simulink model "IDTmodel"  (R2021a)
settings: Solver=ode23tb  StartTime=0.0  StopTime=0.75  FixedStep=4e-4  RelTol=1e-3  EnableMultiTasking=on
PreLoadFcn:
  | % -- Recommended Settings --
  | %
  | %  Simulink:
  | %      Solver: Ode23tb
  | %      Relative tolerance = 1e-4
  | %      Max step size = 0.2
  | %
  | %  Powergui:
  |          Ts = 1e-06; % (discrete electrical model)
  | %
  | %  Control systems:
  |          Ts_control = 10*Ts; % (discrete control system)
  | %
  | % ----------------------------------
InitFcn:
  | Ts=1e-5;
  | Ts_control=1e-5;
undefined symbols (not defined in the file or in its folder): D1, Delta
libraries: spsThreePhaseVIMeasurementLib x26, spsThreePhaseSeriesRLCLoadLib x8, spsabctoAlphaBetaZeroLib x6, spsThreePhaseSeriesRLCBranchLib x6, spsThreePhaseTransformerTwoWindingsLib x5, spsDistributedParametersLineLib x5, spsPowerPositiveSequenceLib x4, spsThreePhaseBreakerLib x4, spsDCVoltageSourceLib x2, spsSVPWMGenerator2LevelLib x2, spsGroundLib x2, spsUniversalBridgeLib x2
(part 2 of 2)

== system IDTmodel/DL-5 ==
  20Km feeder : spsDistributedParametersLineLib/Distributed Parameters Line  Phases=3  Length=20  Frequency=50  Resistance=[0.1153 0.413]  Inductance=[1.05e-3 3.32e-3]  Capacitance=[11.33e-009 5.01e-009]  x1=[-9e-05 -1.85671820461914e-09 0 0;-8e-05 -1.85401382529522e-09 0 0;-7e-05 -1.85129114760334e-09 20803.2327751115 -13139.8661984527;-6e-05 -1.84855019841523e-09 20844.4101545723 -13074.4461801133;-5e-05 -1.84579100478295e-09 20885.3818081202 -13008.8971222685;-4e-05 -1.84301359393864e-09 20926.1473313813 -12943.219671861;-3e-05 -1.8402179932942e-09 20966.7063220166 -12877.4144771007;-2e-05 -1.8374042304411e-09 21007.058379725 -12811.4821874584;-1e-05 -1.83457233315003e-09 21047.2031062481 -12745.4234536591]  x2=[-9e-05 -1.69133325708034e-10 0 0;-8e-05 -1.69244704148608e-10 0 0;-7e-05 -1.69354412212279e-10 20557.5369180313 -13274.4665234826;-6e-05 -1.69462448816273e-10 20599.1383686483 -13209.8177159477;-5e-05 -1.69568812894312e-10 20640.5365140858 -13145.038532845;-4e-05 -1.69673503396625e-10 20681.7309457608 -13080.1296135189;-3e-05 -1.69776519289959e-10 20722.721257101 -13015.0915985941;-2e-05 -1.6987785955759e-10 20763.5070435485 -12949.9251299696;-1e-05 -1.6997752319933e-10 20804.087902564 -12884.6308508122]  x3=[-9e-05 6.18585301934319e-11 0 0;-8e-05 6.20328462935421e-11 0 0;-7e-05 6.22065501545031e-11 37.8134386631987 -16.9223687566623;-6e-05 6.2379640061928e-11 37.8664151634293 -16.8034910224862;-5e-05 6.2552114307489e-11 37.9190179374296 -16.6844474446375;-4e-05 6.27239711889352e-11 37.9712464660314 -16.5652391980283;-3e-05 6.28952090101084e-11 38.0231002337601 -16.4458674591959;-2e-05 6.30658260809605e-11 38.0745787288401 -16.3263334062911;-1e-05 6.32358207175699e-11 38.1256814431994 -16.2066382190668]  x4=[-9e-05 -6.47056572877299e-11 0 0;-8e-05 -6.48780349176388e-11 0 0;-7e-05 -6.50497722275354e-11 96.345814689957 -70.8209858434872;-6e-05 -6.52208675224418e-11 96.5678295656737 -70.5179575504712;-5e-05 -6.53913191137165e-11 96.7888913558986 -70.2142332736835;-4e-05 -6.5561125319071e-11 97.008997878841 -69.9098160107601;-3e-05 -6.57302844625868e-11 97.2281469621385 -69.6047087661763;-2e-05 -6.58987948747313e-11 97.4463364428781 -69.2989145512176;-1e-05 -6.60666548923748e-11 97.6635641676177 -68.9924363839494]  x5=8.1567640642598e-05  V1=[0 0 0 1.943e-09 2.476e+04 2.476e+04;0 0 0 314.2 314.2 314.2;1.571 1.571 1.571 2.213 1.006 -0.5651]  V2=[0 0 0 8.204e-11 2.462e+04 2.462e+04;0 0 0 314.2 314.2 314.2;1.571 1.571 1.571 -1.53 0.9957 -0.5751]  I1=[0 0 0 8.843e-11 41.68 41.68;0 0 0 314.2 314.2 314.2;1.571 1.571 1.571 -2.172 1.148 -0.4225]  I2=[0 0 0 8.932e-11 120.3 120.3;0 0 0 314.2 314.2 314.2;1.571 1.571 1.571 1.001 0.9352 -0.6356]  nHarmo=2  Measurements=None  Decoupling=off  VsMag0=0  VrMag0=0  VsAngle0=0  VrAngle0=0  IsMag0=0  IrMag0=0  IsAngle0=0  IrAngle0=0
      settings: SourceProductBaseCode=PS
  Three-Phase V-I Measurement1 : spsThreePhaseVIMeasurementLib/Three-Phase V-I Measurement  VoltageMeasurement=no  SetLabelV=off  LabelV=Vabc  Vpu=on  VpuLL=off  CurrentMeasurement=no  SetLabelI=off  LabelI=I23  Ipu=on  Pbase=6e6  Vbase=12.47e3  OutputType=Complex  PhasorSimulation=off  PSBequivalent=0
  Three-Phase V-I Measurement4 : spsThreePhaseVIMeasurementLib/Three-Phase V-I Measurement  VoltageMeasurement=no  SetLabelV=off  LabelV=Vabc  Vpu=on  VpuLL=off  CurrentMeasurement=no  SetLabelI=off  LabelI=I23  Ipu=on  Pbase=6e6  Vbase=12.47e3  OutputType=Complex  PhasorSimulation=off  PSBequivalent=0
  A : PMIOPort  Side=Right
  B : PMIOPort  Port=2  Side=Right
  C : PMIOPort  Port=3  Side=Right
  a : PMIOPort  Port=4  Side=Left
  b : PMIOPort  Port=5  Side=Left
  c : PMIOPort  Port=6  Side=Left
  connections:
  c/RConn1 -- Three-Phase V-I Measurement1/LConn3
  a/RConn1 -- Three-Phase V-I Measurement1/LConn1
  b/RConn1 -- Three-Phase V-I Measurement1/LConn2
  A/RConn1 -- Three-Phase V-I Measurement4/LConn1
  B/RConn1 -- Three-Phase V-I Measurement4/LConn2
  C/RConn1 -- Three-Phase V-I Measurement4/LConn3
  20Km feeder/LConn1 -- Three-Phase V-I Measurement4/RConn1
  20Km feeder/LConn2 -- Three-Phase V-I Measurement4/RConn2
  20Km feeder/LConn3 -- Three-Phase V-I Measurement4/RConn3
  20Km feeder/RConn3 -- Three-Phase V-I Measurement1/RConn3
  20Km feeder/RConn1 -- Three-Phase V-I Measurement1/RConn1
  20Km feeder/RConn2 -- Three-Phase V-I Measurement1/RConn2

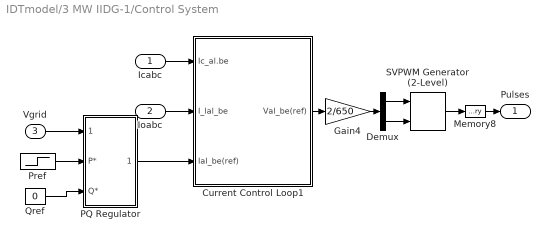
== system IDTmodel/3 MW IIDG-1/Control System ==
  Icabc : Inport
  Ioabc : Inport  Port=2
  Vgrid : Inport  Port=3
  Current Control Loop1 : Subsystem  mask(PR-Controller){Kp=3.5, Wc=pi, Kri=[10 5 2 1]*4, f=50}
      mask prompts: Kp "Propotional Gain(Kp)"; Wc "Cutoff frequency (Wc)"; Kri "Resonant Gains[ki  ki5  ki7  ki11]"; f "Nominal Frequency(f)"
      mask init:
      | Kp=Kp;
      | Ki=Kri(1);
      | Kif=Kri(2);
      | Kis=Kri(3);
      | Kie=Kri(4);
      | f=f;
      | Wc=Wc;
      mask DialogControl Control Prompt: PR-Controller
  Demux : Demux  Outputs=2
  Gain4 : Gain  Gain=2/650
  Memory8 : Memory  InitialCondition=1
  PQ Regulator : Subsystem
  Pref : Step  Before=3000e3  After=3000e3  SampleTime=1e-5
  Qref : Constant  Value=0  VectorParams1D=off  SampleTime=0
  SVPWM Generator (2-Level) : spsSVPWMGenerator2LevelLib/SVPWM Generator (2-Level)  InputType=alpha-beta components  SwitchingPattern=Pattern #1  Fc=9e3  ParUref=[0.8 -30 50]  Ts=1e-5
      settings: SourceProductBaseCode=PS
  Pulses : Outport  VectorParamsAs1DForOutWhenUnconnected=off
  wires:
  Pref/1 -> PQ Regulator/2(P*)
  Qref/1 -> PQ Regulator/3(Q*)
  Demux/2 -> SVPWM Generator (2-Level)/2
  Demux/1 -> SVPWM Generator (2-Level)/1
  Icabc/1 -> Current Control Loop1/1(Ic_al.be)
  Ioabc/1 -> Current Control Loop1/2(I_lal_be)
  Vgrid/1 -> PQ Regulator/1(Val-be)
  PQ Regulator/1(Ial_be*) -> Current Control Loop1/3(Ial_be(ref))
  SVPWM Generator (2-Level)/1 -> Memory8/1
  Gain4/1 -> Demux/1
  Current Control Loop1/1(Val_be(ref)) -> Gain4/1
  Memory8/1 -> Pulses/1

== system IDTmodel/3 MW IIDG-2/Control System ==
  Icabc : Inport
  Ioabc : Inport  Port=2
  Vgrid : Inport  Port=3
  Current Control Loop1 : Subsystem  mask(PR-Controller){Kp=3.5, Wc=pi, Kri=[10 5 2 1]*4, f=50}
      mask prompts: Kp "Propotional Gain(Kp)"; Wc "Cutoff frequency (Wc)"; Kri "Resonant Gains[ki  ki5  ki7  ki11]"; f "Nominal Frequency(f)"
      mask init:
      | Kp=Kp;
      | Ki=Kri(1);
      | Kif=Kri(2);
      | Kis=Kri(3);
      | Kie=Kri(4);
      | f=f;
      | Wc=Wc;
      mask DialogControl Control Prompt: PR-Controller
  Demux : Demux  Outputs=2
  Gain4 : Gain  Gain=2/650
  Memory8 : Memory  InitialCondition=1
  PQ Regulator : Subsystem
  Pref : Step  Before=3000e3  After=3000e3  SampleTime=1e-5
  Qref : Constant  Value=0  VectorParams1D=off  SampleTime=0
  SVPWM Generator (2-Level) : spsSVPWMGenerator2LevelLib/SVPWM Generator (2-Level)  InputType=alpha-beta components  SwitchingPattern=Pattern #1  Fc=9e3  ParUref=[0.8 -30 50]  Ts=1e-5
      settings: SourceProductBaseCode=PS
  Pulses : Outport  VectorParamsAs1DForOutWhenUnconnected=off
  wires:
  Pref/1 -> PQ Regulator/2(P*)
  Qref/1 -> PQ Regulator/3(Q*)
  Demux/2 -> SVPWM Generator (2-Level)/2
  Demux/1 -> SVPWM Generator (2-Level)/1
  Icabc/1 -> Current Control Loop1/1(Ic_al.be)
  Ioabc/1 -> Current Control Loop1/2(I_lal_be)
  Vgrid/1 -> PQ Regulator/1(Val-be)
  PQ Regulator/1(Ial_be*) -> Current Control Loop1/3(Ial_be(ref))
  SVPWM Generator (2-Level)/1 -> Memory8/1
  Gain4/1 -> Demux/1
  Current Control Loop1/1(Val_be(ref)) -> Gain4/1
  Memory8/1 -> Pulses/1

== system IDTmodel/4MVA SG/Regulateurs7 ==
  m : Inport
  Bus Selector1 : BusSelector  OutputSignals="dq0 components.Stator voltage  vq (pu),dq0 components.Stator voltage  vd (pu),Mechanical.Rotor speed  wm  (pu),Output active power   Peo (pu)"
  Math Function1 : Math  Operator=hypot  SignedPower=on  SaturateOnIntegerOverflow=on
  Pref1 : Constant
  Turbine  & Excitation Regulators Mac2 : Subsystem
  Vref : Constant  Value=0.875
  Pm : Outport  VectorParamsAs1DForOutWhenUnconnected=off
  Vf : Outport  Port=2  VectorParamsAs1DForOutWhenUnconnected=off
  wires:
  Pref1/1 -> Turbine  & Excitation Regulators Mac2/2(Vref)
  Turbine  & Excitation Regulators Mac2/1(Pm) -> Pm/1
  Vref/1 -> Turbine  & Excitation Regulators Mac2/1(Pref)
  Turbine  & Excitation Regulators Mac2/2(Vf) -> Vf/1
  Bus Selector1/1 -> Math Function1/1  "<Stator voltage  vq (pu)>"
  Bus Selector1/2 -> Math Function1/2  "<Stator voltage  vd (pu)>"
  Math Function1/1 -> Turbine  & Excitation Regulators Mac2/3(Vm)
  Bus Selector1/3 -> Turbine  & Excitation Regulators Mac2/4(w)  "<Rotor speed  wm  (pu)>"
  Bus Selector1/4 -> Turbine  & Excitation Regulators Mac2/5(Pe)  "<Output active power   Peo (pu)>"
  m/1 -> Bus Selector1/1

== system IDTmodel/4MVA SG1/Regulateurs7 ==
  m : Inport
  Bus Selector1 : BusSelector  OutputSignals="dq0 components.Stator voltage  vq (pu),dq0 components.Stator voltage  vd (pu),Mechanical.Rotor speed  wm  (pu),Output active power   Peo (pu)"
  Math Function1 : Math  Operator=hypot  SignedPower=on  SaturateOnIntegerOverflow=on
  Pref1 : Constant
  Turbine  & Excitation Regulators Mac2 : Subsystem
  Vref : Constant  Value=0.875
  Pm : Outport  VectorParamsAs1DForOutWhenUnconnected=off
  Vf : Outport  Port=2  VectorParamsAs1DForOutWhenUnconnected=off
  wires:
  Pref1/1 -> Turbine  & Excitation Regulators Mac2/2(Vref)
  Turbine  & Excitation Regulators Mac2/1(Pm) -> Pm/1
  Vref/1 -> Turbine  & Excitation Regulators Mac2/1(Pref)
  Turbine  & Excitation Regulators Mac2/2(Vf) -> Vf/1
  Bus Selector1/1 -> Math Function1/1  "<Stator voltage  vq (pu)>"
  Bus Selector1/2 -> Math Function1/2  "<Stator voltage  vd (pu)>"
  Math Function1/1 -> Turbine  & Excitation Regulators Mac2/3(Vm)
  Bus Selector1/3 -> Turbine  & Excitation Regulators Mac2/4(w)  "<Rotor speed  wm  (pu)>"
  Bus Selector1/4 -> Turbine  & Excitation Regulators Mac2/5(Pe)  "<Output active power   Peo (pu)>"
  m/1 -> Bus Selector1/1

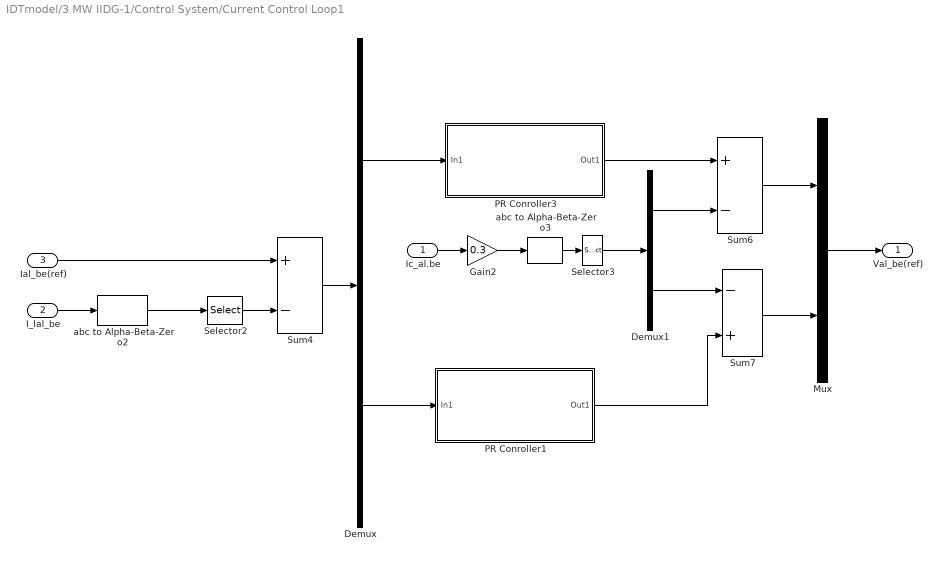
== system IDTmodel/3 MW IIDG-1/Control System/Current Control Loop1 ==
  Ic_al.be : Inport
  I_lal_be : Inport  Port=2
  Ial_be(ref) : Inport  Port=3
  Demux : Demux  Outputs=2
  Demux1 : Demux  Outputs=2
  Gain2 : Gain  Gain=0.3
  Mux : Mux  Inputs=2
  PR Conroller1 : Subsystem
  PR Conroller3 : Subsystem
  Selector2 : Selector  InputPortWidth=3  IndexOptions=Index vector (dialog)  Indices=[1 2]  OutputSizes=1
  Selector3 : Selector  InputPortWidth=3  IndexOptions=Index vector (dialog)  Indices=[1 2]  OutputSizes=1
  Sum4 : Sum  Inputs=+-
  Sum6 : Sum  Inputs=+-
  Sum7 : Sum  Inputs=-+
  abc to Alpha-Beta-Zero2 : spsabctoAlphaBetaZeroLib/abc to Alpha-Beta-Zero
      settings: SourceProductBaseCode=PS
  abc to Alpha-Beta-Zero3 : spsabctoAlphaBetaZeroLib/abc to Alpha-Beta-Zero
      settings: SourceProductBaseCode=PS
  Val_be(ref) : Outport  VectorParamsAs1DForOutWhenUnconnected=off
  wires:
  Selector3/1 -> Demux1/1
  Gain2/1 -> abc to Alpha-Beta-Zero3/1
  abc to Alpha-Beta-Zero3/1 -> Selector3/1
  Demux/2 -> PR Conroller1/1(In1)
  PR Conroller3/1(Out1) -> Sum6/1
  Demux/1 -> PR Conroller3/1(In1)
  Selector2/1 -> Sum4/2
  abc to Alpha-Beta-Zero2/1 -> Selector2/1
  I_lal_be/1 -> abc to Alpha-Beta-Zero2/1
  Sum4/1 -> Demux/1
  Sum7/1 -> Mux/2
  PR Conroller1/1(Out1) -> Sum7/2
  Sum6/1 -> Mux/1
  Demux1/2 -> Sum7/1
  Demux1/1 -> Sum6/2
  Ic_al.be/1 -> Gain2/1
  Mux/1 -> Val_be(ref)/1
  Ial_be(ref)/1 -> Sum4/1

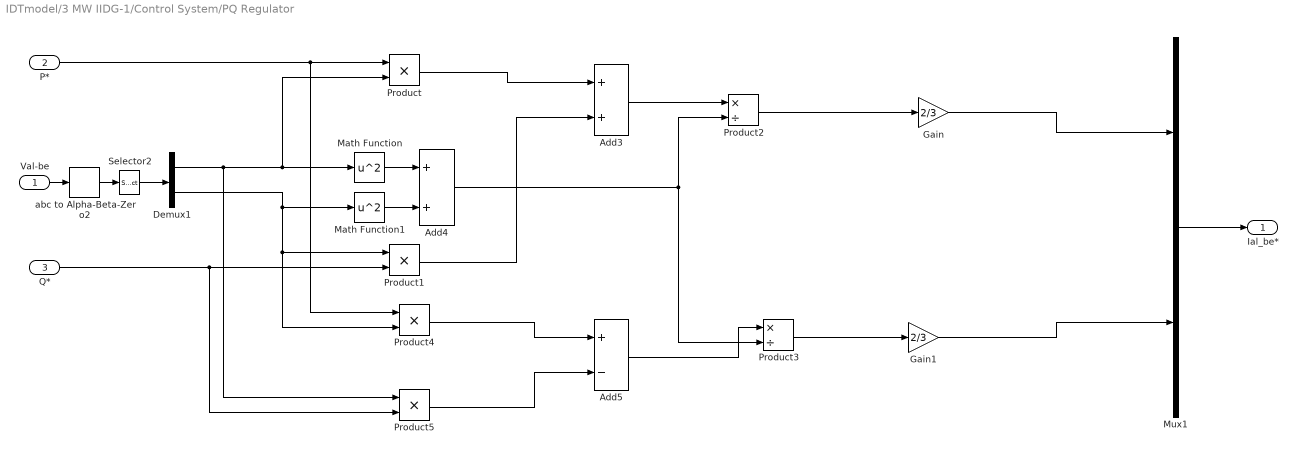
== system IDTmodel/3 MW IIDG-1/Control System/PQ Regulator ==
  Val-be : Inport
  P* : Inport  Port=2
  Q* : Inport  Port=3
  Add3 : Sum
  Add4 : Sum
  Add5 : Sum  Inputs=+-
  Demux1 : Demux  Outputs=2
  Gain : Gain  Gain=2/3
  Gain1 : Gain  Gain=2/3
  Math Function : Math  Operator=square  SignedPower=on  SaturateOnIntegerOverflow=on
  Math Function1 : Math  Operator=square  SignedPower=on  SaturateOnIntegerOverflow=on
  Mux1 : Mux  Inputs=2
  Product{,1,4..5} (4 alike) : Product
  Product2 : Product  Inputs=*/
  Product3 : Product  Inputs=*/
  Selector2 : Selector  InputPortWidth=3  IndexOptions=Index vector (dialog)  Indices=[1 2]  OutputSizes=1
  abc to Alpha-Beta-Zero2 : spsabctoAlphaBetaZeroLib/abc to Alpha-Beta-Zero
      settings: SourceProductBaseCode=PS
  Ial_be* : Outport  VectorParamsAs1DForOutWhenUnconnected=off
  wires:
  Val-be/1 -> abc to Alpha-Beta-Zero2/1
  abc to Alpha-Beta-Zero2/1 -> Selector2/1
  Product5/1 -> Add5/2
  Product4/1 -> Add5/1
  Gain1/1 -> Mux1/2
  Product3/1 -> Gain1/1
  Gain/1 -> Mux1/1
  Product2/1 -> Gain/1
  Add5/1 -> Product3/1
  Add4/1 -> Product2/2, Product3/2
  Add3/1 -> Product2/1
  Math Function1/1 -> Add4/2
  Math Function/1 -> Add4/1
  Product1/1 -> Add3/2
  Product/1 -> Add3/1
  Demux1/2 -> Product1/1, Product4/2, Math Function1/1
  Demux1/1 -> Math Function/1, Product/2, Product5/1
  Selector2/1 -> Demux1/1
  Mux1/1 -> Ial_be*/1
  Q*/1 -> Product1/2, Product5/2
  P*/1 -> Product/1, Product4/1

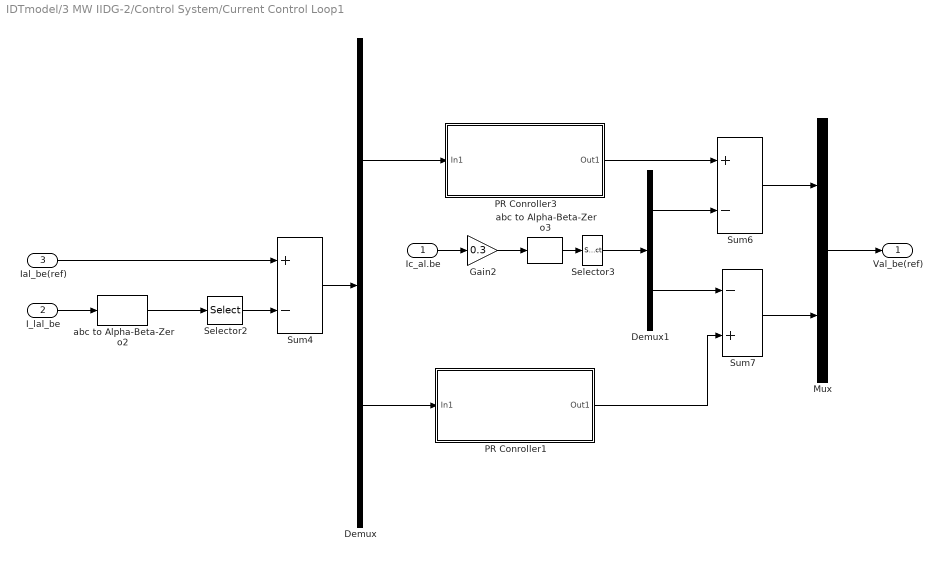
== system IDTmodel/3 MW IIDG-2/Control System/Current Control Loop1 ==
  Ic_al.be : Inport
  I_lal_be : Inport  Port=2
  Ial_be(ref) : Inport  Port=3
  Demux : Demux  Outputs=2
  Demux1 : Demux  Outputs=2
  Gain2 : Gain  Gain=0.3
  Mux : Mux  Inputs=2
  PR Conroller1 : Subsystem
  PR Conroller3 : Subsystem
  Selector2 : Selector  InputPortWidth=3  IndexOptions=Index vector (dialog)  Indices=[1 2]  OutputSizes=1
  Selector3 : Selector  InputPortWidth=3  IndexOptions=Index vector (dialog)  Indices=[1 2]  OutputSizes=1
  Sum4 : Sum  Inputs=+-
  Sum6 : Sum  Inputs=+-
  Sum7 : Sum  Inputs=-+
  abc to Alpha-Beta-Zero2 : spsabctoAlphaBetaZeroLib/abc to Alpha-Beta-Zero
      settings: SourceProductBaseCode=PS
  abc to Alpha-Beta-Zero3 : spsabctoAlphaBetaZeroLib/abc to Alpha-Beta-Zero
      settings: SourceProductBaseCode=PS
  Val_be(ref) : Outport  VectorParamsAs1DForOutWhenUnconnected=off
  wires:
  Selector3/1 -> Demux1/1
  Gain2/1 -> abc to Alpha-Beta-Zero3/1
  abc to Alpha-Beta-Zero3/1 -> Selector3/1
  Demux/2 -> PR Conroller1/1(In1)
  PR Conroller3/1(Out1) -> Sum6/1
  Demux/1 -> PR Conroller3/1(In1)
  Selector2/1 -> Sum4/2
  abc to Alpha-Beta-Zero2/1 -> Selector2/1
  I_lal_be/1 -> abc to Alpha-Beta-Zero2/1
  Sum4/1 -> Demux/1
  Sum7/1 -> Mux/2
  PR Conroller1/1(Out1) -> Sum7/2
  Sum6/1 -> Mux/1
  Demux1/2 -> Sum7/1
  Demux1/1 -> Sum6/2
  Ic_al.be/1 -> Gain2/1
  Mux/1 -> Val_be(ref)/1
  Ial_be(ref)/1 -> Sum4/1

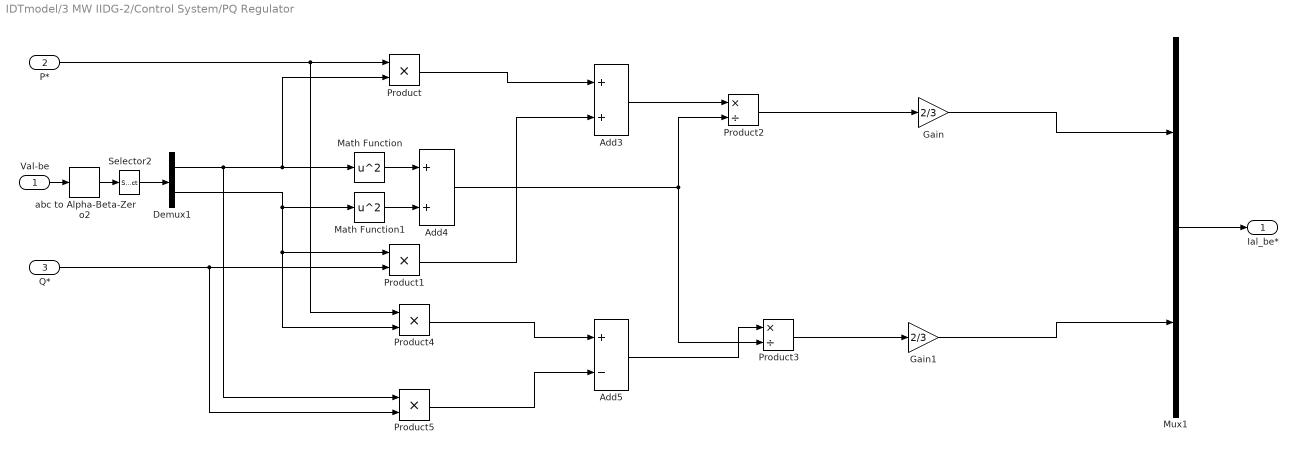
== system IDTmodel/3 MW IIDG-2/Control System/PQ Regulator ==
  Val-be : Inport
  P* : Inport  Port=2
  Q* : Inport  Port=3
  Add3 : Sum
  Add4 : Sum
  Add5 : Sum  Inputs=+-
  Demux1 : Demux  Outputs=2
  Gain : Gain  Gain=2/3
  Gain1 : Gain  Gain=2/3
  Math Function : Math  Operator=square  SignedPower=on  SaturateOnIntegerOverflow=on
  Math Function1 : Math  Operator=square  SignedPower=on  SaturateOnIntegerOverflow=on
  Mux1 : Mux  Inputs=2
  Product{,1,4..5} (4 alike) : Product
  Product2 : Product  Inputs=*/
  Product3 : Product  Inputs=*/
  Selector2 : Selector  InputPortWidth=3  IndexOptions=Index vector (dialog)  Indices=[1 2]  OutputSizes=1
  abc to Alpha-Beta-Zero2 : spsabctoAlphaBetaZeroLib/abc to Alpha-Beta-Zero
      settings: SourceProductBaseCode=PS
  Ial_be* : Outport  VectorParamsAs1DForOutWhenUnconnected=off
  wires:
  Val-be/1 -> abc to Alpha-Beta-Zero2/1
  abc to Alpha-Beta-Zero2/1 -> Selector2/1
  Product5/1 -> Add5/2
  Product4/1 -> Add5/1
  Gain1/1 -> Mux1/2
  Product3/1 -> Gain1/1
  Gain/1 -> Mux1/1
  Product2/1 -> Gain/1
  Add5/1 -> Product3/1
  Add4/1 -> Product2/2, Product3/2
  Add3/1 -> Product2/1
  Math Function1/1 -> Add4/2
  Math Function/1 -> Add4/1
  Product1/1 -> Add3/2
  Product/1 -> Add3/1
  Demux1/2 -> Product1/1, Product4/2, Math Function1/1
  Demux1/1 -> Math Function/1, Product/2, Product5/1
  Selector2/1 -> Demux1/1
  Mux1/1 -> Ial_be*/1
  Q*/1 -> Product1/2, Product5/2
  P*/1 -> Product/1, Product4/1

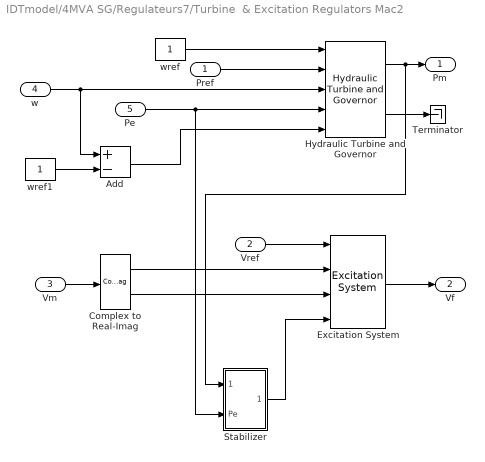
== system IDTmodel/4MVA SG/Regulateurs7/Turbine  & Excitation Regulators Mac2 ==
  Pref : Inport
  Vref : Inport  Port=2
  Vm : Inport  Port=3
  w : Inport  Port=4
  Pe : Inport  Port=5
  Add : Sum  Inputs=+-
  Complex to Real-Imag : ComplexToRealImag
  Excitation System : spsExcitationSystemLib/Excitation System  tr=20e-3  reg=[ 30, 0.001 ]  exc=[ 1, 0 ]  tgr=[ 0, 0 ]  damp=[ 0.001, 0.1 ]  sat=[ 0, 0 ]  lim=[ -11.5, 11.5, 0 ]  v0=[1,1.8534]
      settings: SourceProductBaseCode=PS
  Hydraulic Turbine and Governor : spsHydraulicTurbineandGovernorLib/Hydraulic Turbine and Governor  sm="[ 10/3  0.07 ]"  gate="[  0.01  0.97518  -0.1  0.1 ]"  reg="[  0.005 0.9163  0.105  0  0.01  ]"  hyd="[  0  2.67  ]"  dref=0  po=0.882339
      settings: SourceProductBaseCode=PS
  Stabilizer : Subsystem
  Terminator : Terminator
  wref : Constant
  wref1 : Constant
  Pm : Outport  VectorParamsAs1DForOutWhenUnconnected=off
  Vf : Outport  Port=2  VectorParamsAs1DForOutWhenUnconnected=off
  wires:
  Hydraulic Turbine and Governor/2 -> Terminator/1
  Hydraulic Turbine and Governor/1 -> Pm/1, Stabilizer/1(Pm)
  Excitation System/1 -> Vf/1
  Pe/1 -> Hydraulic Turbine and Governor/4, Stabilizer/2(Pe)
  Pref/1 -> Hydraulic Turbine and Governor/2
  Vref/1 -> Excitation System/1
  wref/1 -> Hydraulic Turbine and Governor/1
  w/1 -> Hydraulic Turbine and Governor/3, Add/1
  Vm/1 -> Complex to Real-Imag/1
  Complex to Real-Imag/2 -> Excitation System/3
  Complex to Real-Imag/1 -> Excitation System/2
  wref1/1 -> Add/2
  Add/1 -> Hydraulic Turbine and Governor/5
  Stabilizer/1(Stab) -> Excitation System/4

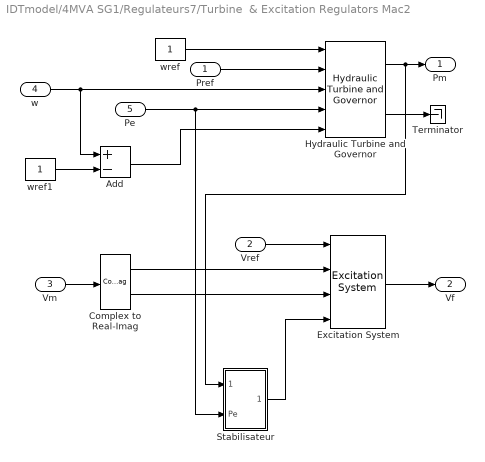
== system IDTmodel/4MVA SG1/Regulateurs7/Turbine  & Excitation Regulators Mac2 ==
  Pref : Inport
  Vref : Inport  Port=2
  Vm : Inport  Port=3
  w : Inport  Port=4
  Pe : Inport  Port=5
  Add : Sum  Inputs=+-
  Complex to Real-Imag : ComplexToRealImag
  Excitation System : spsExcitationSystemLib/Excitation System  tr=20e-3  reg=[ 30, 0.001 ]  exc=[ 1, 0 ]  tgr=[ 0, 0 ]  damp=[ 0.001, 0.1 ]  sat=[ 0, 0 ]  lim=[ -11.5, 11.5, 0 ]  v0=[1,1.84636]
      settings: SourceProductBaseCode=PS
  Hydraulic Turbine and Governor : spsHydraulicTurbineandGovernorLib/Hydraulic Turbine and Governor  sm="[ 10/3  0.07 ]"  gate="[  0.01  0.97518  -0.1  0.1 ]"  reg="[  0.005 0.9163  0.105  0  0.01  ]"  hyd="[  0  2.67  ]"  dref=0  po=0.882168
      settings: SourceProductBaseCode=PS
  Stabilisateur : Subsystem
  Terminator : Terminator
  wref : Constant
  wref1 : Constant
  Pm : Outport  VectorParamsAs1DForOutWhenUnconnected=off
  Vf : Outport  Port=2  VectorParamsAs1DForOutWhenUnconnected=off
  wires:
  Hydraulic Turbine and Governor/2 -> Terminator/1
  Hydraulic Turbine and Governor/1 -> Pm/1, Stabilisateur/1(Pm)
  Excitation System/1 -> Vf/1
  Pe/1 -> Hydraulic Turbine and Governor/4, Stabilisateur/2(Pe)
  Pref/1 -> Hydraulic Turbine and Governor/2
  Vref/1 -> Excitation System/1
  wref/1 -> Hydraulic Turbine and Governor/1
  w/1 -> Hydraulic Turbine and Governor/3, Add/1
  Vm/1 -> Complex to Real-Imag/1
  Complex to Real-Imag/2 -> Excitation System/3
  Complex to Real-Imag/1 -> Excitation System/2
  wref1/1 -> Add/2
  Add/1 -> Hydraulic Turbine and Governor/5
  Stabilisateur/1(Stab) -> Excitation System/4

== system IDTmodel/3 MW IIDG-1/Control System/Current Control Loop1/PR Conroller1 ==
  In1 : Inport
  Gain : Gain  Gain=Kp
  Sum2 : Sum  Inputs=+++++
  Transfer Fcn2 : TransferFcn  Numerator=[2*Kif*Wc 0]  Denominator=[1 0 (2*pi*f)^2]
  Transfer Fcn21 : TransferFcn  Numerator=[2*Ki*Wc 0]  Denominator=[1 0 (2*pi*f)^2]
  Transfer Fcn3 : TransferFcn  Numerator=[2*Kis*Wc 0]  Denominator=[1 0 (2*pi*f)^2]
  Transfer Fcn4 : TransferFcn  Numerator=[2*Kie*Wc 0]  Denominator=[1 0 (2*pi*f)^2]
  Out1 : Outport  VectorParamsAs1DForOutWhenUnconnected=off
  wires:
  Transfer Fcn3/1 -> Sum2/4
  Transfer Fcn21/1 -> Sum2/2
  In1/1 -> Transfer Fcn4/1, Transfer Fcn2/1, Gain/1, Transfer Fcn21/1, Transfer Fcn3/1
  Gain/1 -> Sum2/1
  Sum2/1 -> Out1/1
  Transfer Fcn4/1 -> Sum2/5
  Transfer Fcn2/1 -> Sum2/3

== system IDTmodel/3 MW IIDG-1/Control System/Current Control Loop1/PR Conroller3 ==
  In1 : Inport
  Gain : Gain  Gain=Kp
  Sum2 : Sum  Inputs=+++++
  Transfer Fcn2 : TransferFcn  Numerator=[2*Kif*Wc 0]  Denominator=[1 0 (2*pi*f)^2]
  Transfer Fcn21 : TransferFcn  Numerator=[2*Ki*Wc 0]  Denominator=[1 0 (2*pi*f)^2]
  Transfer Fcn3 : TransferFcn  Numerator=[2*Kis*Wc 0]  Denominator=[1 0 (2*pi*f)^2]
  Transfer Fcn4 : TransferFcn  Numerator=[2*Kie*Wc 0]  Denominator=[1 0 (2*pi*f)^2]
  Out1 : Outport  VectorParamsAs1DForOutWhenUnconnected=off
  wires:
  Transfer Fcn2/1 -> Sum2/3
  Transfer Fcn4/1 -> Sum2/5
  Sum2/1 -> Out1/1
  Gain/1 -> Sum2/1
  In1/1 -> Transfer Fcn3/1, Transfer Fcn21/1, Gain/1, Transfer Fcn2/1, Transfer Fcn4/1
  Transfer Fcn21/1 -> Sum2/2
  Transfer Fcn3/1 -> Sum2/4

== system IDTmodel/3 MW IIDG-2/Control System/Current Control Loop1/PR Conroller1 ==
  In1 : Inport
  Gain : Gain  Gain=Kp
  Sum2 : Sum  Inputs=+++++
  Transfer Fcn2 : TransferFcn  Numerator=[2*Kif*Wc 0]  Denominator=[1 0 (2*pi*f)^2]
  Transfer Fcn21 : TransferFcn  Numerator=[2*Ki*Wc 0]  Denominator=[1 0 (2*pi*f)^2]
  Transfer Fcn3 : TransferFcn  Numerator=[2*Kis*Wc 0]  Denominator=[1 0 (2*pi*f)^2]
  Transfer Fcn4 : TransferFcn  Numerator=[2*Kie*Wc 0]  Denominator=[1 0 (2*pi*f)^2]
  Out1 : Outport  VectorParamsAs1DForOutWhenUnconnected=off
  wires:
  Transfer Fcn3/1 -> Sum2/4
  Transfer Fcn21/1 -> Sum2/2
  In1/1 -> Transfer Fcn4/1, Transfer Fcn2/1, Gain/1, Transfer Fcn21/1, Transfer Fcn3/1
  Gain/1 -> Sum2/1
  Sum2/1 -> Out1/1
  Transfer Fcn4/1 -> Sum2/5
  Transfer Fcn2/1 -> Sum2/3

== system IDTmodel/3 MW IIDG-2/Control System/Current Control Loop1/PR Conroller3 ==
  In1 : Inport
  Gain : Gain  Gain=Kp
  Sum2 : Sum  Inputs=+++++
  Transfer Fcn2 : TransferFcn  Numerator=[2*Kif*Wc 0]  Denominator=[1 0 (2*pi*f)^2]
  Transfer Fcn21 : TransferFcn  Numerator=[2*Ki*Wc 0]  Denominator=[1 0 (2*pi*f)^2]
  Transfer Fcn3 : TransferFcn  Numerator=[2*Kis*Wc 0]  Denominator=[1 0 (2*pi*f)^2]
  Transfer Fcn4 : TransferFcn  Numerator=[2*Kie*Wc 0]  Denominator=[1 0 (2*pi*f)^2]
  Out1 : Outport  VectorParamsAs1DForOutWhenUnconnected=off
  wires:
  Transfer Fcn2/1 -> Sum2/3
  Transfer Fcn4/1 -> Sum2/5
  Sum2/1 -> Out1/1
  Gain/1 -> Sum2/1
  In1/1 -> Transfer Fcn3/1, Transfer Fcn21/1, Gain/1, Transfer Fcn2/1, Transfer Fcn4/1
  Transfer Fcn21/1 -> Sum2/2
  Transfer Fcn3/1 -> Sum2/4

== system IDTmodel/4MVA SG/Regulateurs7/Turbine  & Excitation Regulators Mac2/Stabilizer ==
  Pm : Inport
  Pe : Inport  Port=2
  Generic Power System Stabilizer : spsGenericPowerSystemStabilizerLib/Generic Power System Stabilizer  Tsensor=15e-3  K=2.5  Twashout=1  Tleadlag1="[0.06  1]"  Tleadlag2="[0  0]"  VSlimits=[-0.15 0.15]  Vinit=0  Plot_On=off  MagdB_On=on  FreqRange=logspace(-2,2,500)
      settings: SourceProductBaseCode=PS
  Sum2 : Sum  Inputs=+-  InputSameDT=on  SaturateOnIntegerOverflow=on  OutDataTypeStr=Inherit: Same as first input
  Stab : Outport  InitialOutput=0  VectorParamsAs1DForOutWhenUnconnected=off
  wires:
  Generic Power System Stabilizer/1 -> Stab/1
  Sum2/1 -> Generic Power System Stabilizer/1
  Pm/1 -> Sum2/1
  Pe/1 -> Sum2/2

== system IDTmodel/4MVA SG1/Regulateurs7/Turbine  & Excitation Regulators Mac2/Stabilisateur ==
  Pm : Inport
  Pe : Inport  Port=2
  Generic Power System Stabilizer : spsGenericPowerSystemStabilizerLib/Generic Power System Stabilizer  Tsensor=15e-3  K=2.5  Twashout=1  Tleadlag1="[0.06  1]"  Tleadlag2="[0  0]"  VSlimits=[-0.15 0.15]  Vinit=0  Plot_On=off  MagdB_On=on  FreqRange=logspace(-2,2,500)
      settings: SourceProductBaseCode=PS
  Sum2 : Sum  Inputs=+-  InputSameDT=on  SaturateOnIntegerOverflow=on  OutDataTypeStr=Inherit: Same as first input
  Stab : Outport  InitialOutput=0  VectorParamsAs1DForOutWhenUnconnected=off
  wires:
  Generic Power System Stabilizer/1 -> Stab/1
  Sum2/1 -> Generic Power System Stabilizer/1
  Pm/1 -> Sum2/1
  Pe/1 -> Sum2/2
